simulink model "control_on_off"  (R2020b)
settings: Solver=VariableStepAuto  StartTime=0.0  StopTime=50  RelTol=1e-3
settings Model: Creator=Acer  LastModifiedBy=Acer

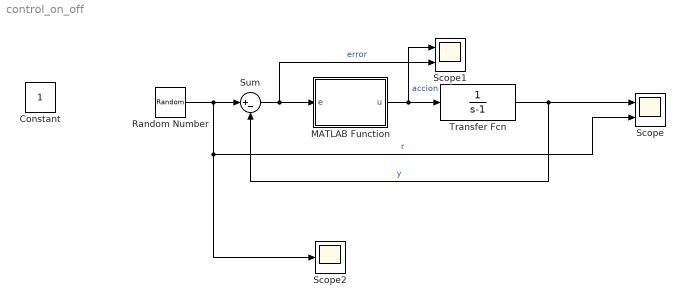
== system control_on_off ==
  Constant : Constant
  MATLAB Function : MATLAB Function  TreatAsAtomicUnit=on
  Random Number : RandomNumber  SampleTime=7
  Scope : Scope  NumInputPorts=2
  Scope1 : Scope  NumInputPorts=2
  Scope2 : Scope
  Sum : Sum  Inputs=|+-
  Transfer Fcn : TransferFcn  Denominator=[1 -1]
  wires:
  Transfer Fcn/1 -> Scope/1, Sum/2  "y"
  Sum/1 -> Scope1/2, MATLAB Function/1(e)  "error"
  MATLAB Function/1(u) -> Scope1/1, Transfer Fcn/1  "accion"
  Random Number/1 -> Scope/2, Scope2/1, Sum/1  "r"

== matlab function control_on_off/MATLAB Function ==
  data: e input; u output
function u = cont_on_off(e)
if e>=0
    u=1;
else
    u=0;
end
